simulink model "Googol_XY_machine_test"  (R2020a)
settings: Solver=ode14x  StartTime=0.0  StopTime=15  RelTol=1e-3  EnableMultiTasking=on
values from neighbouring files (symbols this model uses):
  N = length(signal)    [plotfft.m]    (also in script_cascade.m = length(out_with.cascade.signals(2).values); script_pid.m = length(out_with.PID.signals(2).values))
  new_kd = gains(1)    [script.m]    (also in script_pid.m)
  new_ki = gains(3)    [script.m]    (also in script_pid.m)
  new_kp = gains(2)    [script.m]    (also in script_pid.m)
undefined symbols (not defined in the file or in its folder): X, Y, Z
libraries: sm_lib x10, simulink x8, nesl_utility x7
settings Model: Creator=Admin  LastModifiedBy=Admin
settings SolverCC: AutoInsertRateTranBlk=on
settings DataIOCC: LimitDataPoints=on  MaxDataPoints=10000  ReturnWorkspaceOutputsName=out_without
settings OptimizationCC: LifeSpan=inf
settings DebuggingCC: AllowSymbolicDim=off  SFUnexpectedBacktrackingDiag=warning  SFNoUnconditionalDefaultTransitionDiag=warning  SFExecutionAtInitializationDiag=none  ArithmeticOperatorsInVariantConditions=warning
settings SFSimCC: SimUseLocalCustomCode=off  CustomCodeUndefinedFunction=UseInterfaceOnly
settings RTWCC: RTWUseLocalCustomCode=off
settings CodeAppCC: StateflowObjectComments=on
settings GRTTargetCC: TargetLangStandard=C89/C90 (ANSI)
settings ConfigComp: CovMetricSettings=dw  CovHtmlReporting=on  CovSaveCumulativeToWorkspaceVar=on  CovSaveSingleToWorkspaceVar=on  CovExternalEMLEnable=off  CovSFcnEnable=off
settings SimscapeCC: SimscapeLogType=all  SimscapeLogSimulationStatistics=on  SimscapeLogDataHistory=10000

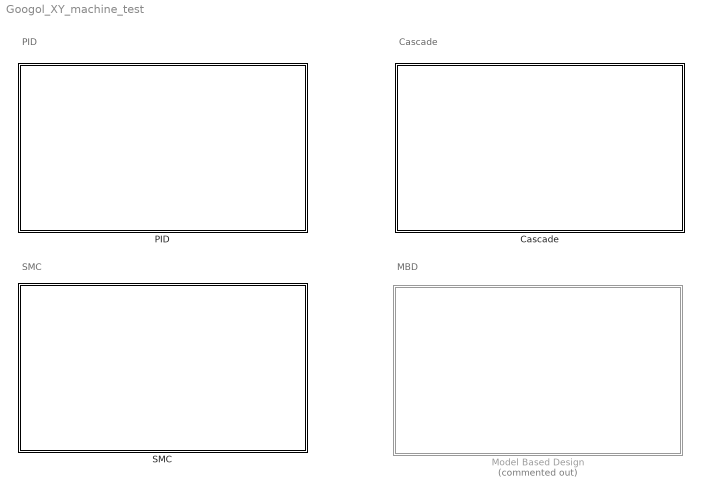
== system Googol_XY_machine_test ==
  note: MBD
  note: Cascade
  note: PID
  note: SMC
  Cascade : Subsystem
  Model Based Design : Subsystem  Commented=on
  PID : Subsystem
  SMC : Subsystem

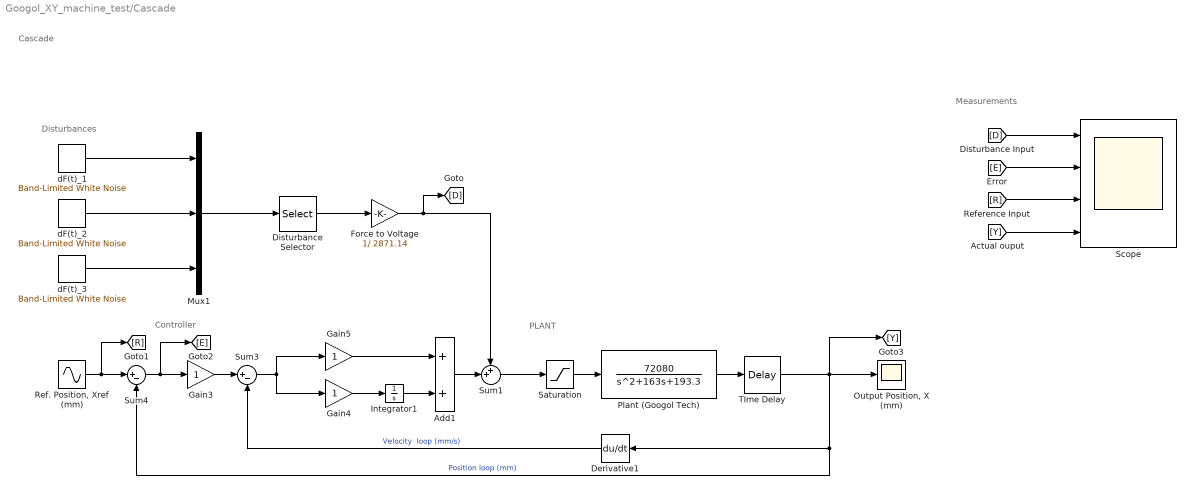
== system Googol_XY_machine_test/Cascade ==
  note: PLANT
  note: Controller
  note: Measurements
  note: Disturbances
  note: Cascade
  Add1 : Sum
  Derivative1 : Derivative
  Disturbance Selector : Selector  InputPortWidth=3  IndexOptions=Index vector (dialog)  Indices=[1]  OutputSizes=1
  Force to Voltage : Gain  Gain=1/ 2871.14
  Gain3 : Gain
  Gain4 : Gain
  Gain5 : Gain
  Integrator1 : Integrator  InitialCondition=.1
  Mux1 : Mux  Inputs=3
  "Output Position, X (mm)" : Scope
  Plant (Googol Tech) : TransferFcn  Numerator=[72080]  Denominator=[1 163 193.3]
  "Ref. Position, Xref (mm)" : Sin  SampleTime=0
  Saturation : Saturate  UpperLimit=92  LowerLimit=-92
  Scope : Scope  NumInputPorts=4
  Sum1 : Sum  Inputs=++|
  Sum3 : Sum  Inputs=|+-
  Sum4 : Sum  Inputs=|+-
  TIme Delay : TransportDelay  DelayTime=0.0012
  dF(t)_1 : simulink/Sources/Band-Limited White Noise  Cov=[0.1]  Ts=5e-4  seed=[23341]
  dF(t)_2 : simulink/Sources/Band-Limited White Noise  Cov=[0.1]  Ts=0.1  seed=[23341]
  dF(t)_3 : simulink/Sources/Band-Limited White Noise  Cov=[0.1]  Ts=0.1  seed=[23341]
  wires:
  dF(t)_3/1 -> Mux1/3
  TIme Delay/1 -> "Output Position, X (mm)"/1, [Y], Derivative1/1, Sum4/2  "Position loop (mm)"
  Sum1/1 -> Saturation/1
  Gain5/1 -> Add1/1
  Integrator1/1 -> Add1/2
  Plant (Googol Tech)/1 -> TIme Delay/1
  Sum3/1 -> Gain5/1, Gain4/1
  "Ref. Position, Xref (mm)"/1 -> Sum4/1, [R]
  Sum4/1 -> Gain3/1, [E]
  Derivative1/1 -> Sum3/2  "Velocity  loop (mm/s)"
  Gain3/1 -> Sum3/1
  Disturbance Selector/1 -> Force to Voltage/1
  Gain4/1 -> Integrator1/1
  Add1/1 -> Sum1/2
  dF(t)_2/1 -> Mux1/2
  dF(t)_1/1 -> Mux1/1
  Mux1/1 -> Disturbance Selector/1
  Force to Voltage/1 -> Sum1/1, [D]
  [D] -> Scope/1
  [E] -> Scope/2
  [R] -> Scope/3
  [Y] -> Scope/4
  Saturation/1 -> Plant (Googol Tech)/1

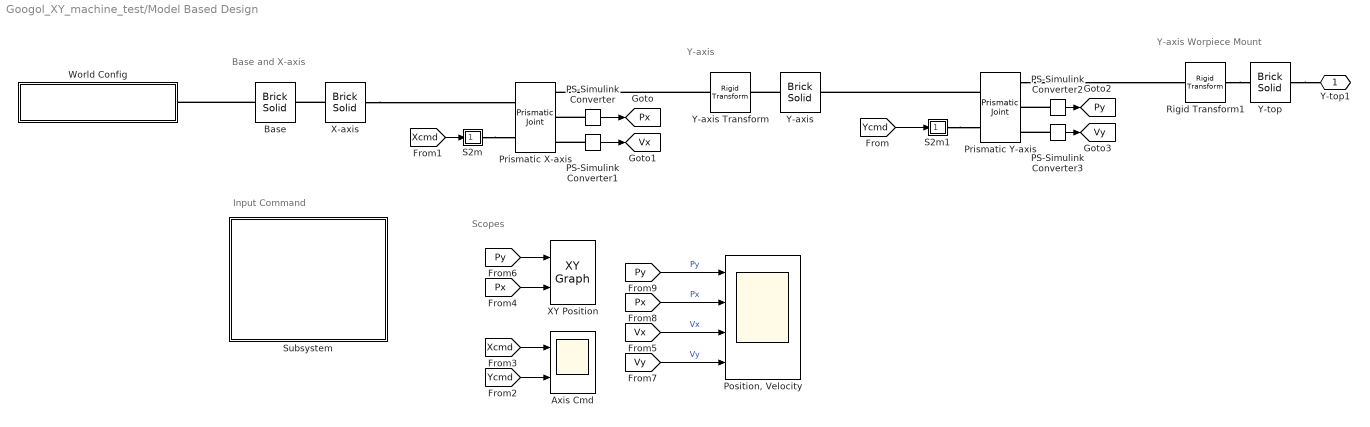
== system Googol_XY_machine_test/Model Based Design ==
  note: Input Command
  note: Scopes
  note: Base and X-axis
  note: Y-axis
  note: Y-axis Worpiece Mount
  Axis Cmd : Scope  NumInputPorts=2
  Base : sm_lib/Body Elements/Brick Solid  GraphicAmbientColor=[0.15 0.15 0.15 1.0]  BasedOnType=Density  BrickDimensions=[630 470 10]  BrickDimensionUnits=mm  CenterOfMass=[0 0 0]  CenterOfMassUnits=m  GraphicDiffuseColor=[0.4 0.4 0.4]  Density=1000  DensityUnits=kg/m^3  DoExposeReferenceFrame=on  GraphicEmissiveColor=[0.0 0.0 0.0 1.0]  ExportEntireGeometry=off  SerializedFrames=<Frames><Frame><Id>Frame1</Id><Value><Name>F1</Name><Origin><Source>GeometricFeature</Source><FeatureName>+z surface</FeatureName></Origin><PrimaryAxis><DefinedDirection>+Z</DefinedDirection><Source>ReferenceFrame</Source><SourceDirection>+Z</SourceDirection><FeatureName></FeatureName></PrimaryAxis><SecondaryAxis><DefinedDirection>+X</DefinedDirection><Source>ReferenceFrame</Source><SourceDirection>+X</SourceDirection><FeatureName></FeatureName></SecondaryAxis></Value></Frame></Frames>  MarkerShape=Sphere  MarkerSize=10  GraphicType=FromGeometry  InertiaType=CalculateFromGeometry  Mass=1  MassUnits=kg  MomentsOfInertia=[1 1 1]  MomentsOfInertiaUnits=kg*m^2  GraphicOpacity=1.0  ProductsOfInertia=[0 0 0]  ProductsOfInertiaUnits=kg*m^2  GraphicShininess=75  GraphicSpecularColor=[0.5 0.5 0.5 1.0]  GraphicVisPropType=SimpleVisualProperties
  PS-Simulink Converter : nesl_utility/PS-Simulink Converter  PhysicalDomain=network_engine_domain  SubClassName=ps_output  LeftPortType=input  RightPortType=output  PseudoPeriodic=off  Frequencies=[]  Unit=mm  AffineConversion=off
  PS-Simulink Converter1 : nesl_utility/PS-Simulink Converter  PhysicalDomain=network_engine_domain  SubClassName=ps_output  LeftPortType=input  RightPortType=output  PseudoPeriodic=off  Frequencies=[]  Unit=m/s  AffineConversion=off
  PS-Simulink Converter2 : nesl_utility/PS-Simulink Converter  PhysicalDomain=network_engine_domain  SubClassName=ps_output  LeftPortType=input  RightPortType=output  PseudoPeriodic=off  Frequencies=[]  Unit=mm  AffineConversion=off
  PS-Simulink Converter3 : nesl_utility/PS-Simulink Converter  PhysicalDomain=network_engine_domain  SubClassName=ps_output  LeftPortType=input  RightPortType=output  PseudoPeriodic=off  Frequencies=[]  Unit=m/s  AffineConversion=off
  "Position, Velocity" : Scope  NumInputPorts=4
  Prismatic X-axis : sm_lib/Joints/Prismatic Joint  JointMode=Normal  SenseConstraintForce=off  SenseConstraintForceX=off  SenseConstraintForceY=off  SenseConstraintForceZ=off  SenseConstraintTorque=off  SenseConstraintTorqueX=off  SenseConstraintTorqueY=off  SenseConstraintTorqueZ=off  SenseTotalForce=off  SenseTotalForceX=off  SenseTotalForceY=off  SenseTotalForceZ=off  SenseTotalTorque=off  SenseTotalTorqueX=off  SenseTotalTorqueY=off  SenseTotalTorqueZ=off  CompositeWrenchDir=FollowerOnBase  CompositeWrenchFrame=BaseFrame  EquilibriumPosition=0  EquilibriumPositionUnits=m  SpringStiffness=0  SpringStiffnessUnits=N/m  DampingCoefficient=0  DampingCoefficientUnits=N/(m/s)  TorqueActuationMode=ComputedTorque  MotionActuationMode=InputMotion  SensePosition=on  SenseVelocity=on  SenseAcceleration=off  SenseTorqueForce=off  SenseLowerLimitTorqueForce=off  SenseUpperLimitTorqueForce=off  LowerLimitSpecify=on  LowerLimitBound=-115  LowerLimitBoundUnits=mm  LowerLimitStiffness=1e3  LowerLimitStiffnessUnits=N/m  LowerLimitDamping=1e3  LowerLimitDampingUnits=N/(m/s)  LowerLimitTransitionRegionWidth=1e-4  LowerLimitTransitionRegionWidthUnits=m  UpperLimitSpecify=on  UpperLimitBound=115  UpperLimitBoundUnits=mm  UpperLimitStiffness=1e3  UpperLimitStiffnessUnits=N/m  UpperLimitDamping=1e3  UpperLimitDampingUnits=N/(m/s)  UpperLimitTransitionRegionWidth=1e-4  UpperLimitTransitionRegionWidthUnits=m  PositionTargetSpecify=off  PositionTargetPriority=High  PositionTargetValue=0  PositionTargetValueUnits=m  VelocityTargetSpecify=off  VelocityTargetPriority=High  VelocityTargetValue=0  VelocityTargetValueUnits=m/s
  Prismatic Y-axis : sm_lib/Joints/Prismatic Joint  JointMode=Normal  SenseConstraintForce=off  SenseConstraintForceX=off  SenseConstraintForceY=off  SenseConstraintForceZ=off  SenseConstraintTorque=off  SenseConstraintTorqueX=off  SenseConstraintTorqueY=off  SenseConstraintTorqueZ=off  SenseTotalForce=off  SenseTotalForceX=off  SenseTotalForceY=off  SenseTotalForceZ=off  SenseTotalTorque=off  SenseTotalTorqueX=off  SenseTotalTorqueY=off  SenseTotalTorqueZ=off  CompositeWrenchDir=FollowerOnBase  CompositeWrenchFrame=BaseFrame  EquilibriumPosition=0  EquilibriumPositionUnits=m  SpringStiffness=0  SpringStiffnessUnits=N/m  DampingCoefficient=0  DampingCoefficientUnits=N/(m/s)  TorqueActuationMode=ComputedTorque  MotionActuationMode=InputMotion  SensePosition=on  SenseVelocity=on  SenseAcceleration=off  SenseTorqueForce=off  SenseLowerLimitTorqueForce=off  SenseUpperLimitTorqueForce=off  LowerLimitSpecify=on  LowerLimitBound=-115  LowerLimitBoundUnits=mm  LowerLimitStiffness=10  LowerLimitStiffnessUnits=N/m  LowerLimitDamping=1e3  LowerLimitDampingUnits=N/(m/s)  LowerLimitTransitionRegionWidth=1e-4  LowerLimitTransitionRegionWidthUnits=m  UpperLimitSpecify=on  UpperLimitBound=115  UpperLimitBoundUnits=mm  UpperLimitStiffness=10  UpperLimitStiffnessUnits=N/m  UpperLimitDamping=1e3  UpperLimitDampingUnits=N/(m/s)  UpperLimitTransitionRegionWidth=1e-4  UpperLimitTransitionRegionWidthUnits=m  PositionTargetSpecify=off  PositionTargetPriority=High  PositionTargetValue=0  PositionTargetValueUnits=m  VelocityTargetSpecify=off  VelocityTargetPriority=High  VelocityTargetValue=0  VelocityTargetValueUnits=m/s
  Rigid Transform1 : sm_lib/Frames and Transforms/Rigid Transform  TranslationMethod=None  TranslationStandardOffset=0  TranslationLengthUnit=m  TranslationStandardAxis=+Z  TranslationCartesianOffset=[0 0 0]  TranslationROffset=0  TranslationROffsetUnits=m  TranslationZOffset=0  TranslationZOffsetUnits=m  TranslationThetaOffset=0  TranslationThetaOffsetUnits=deg  RotationMethod=StandardAxis  RotationAngleUnits=deg  RotationStandardAxis=+Y  RotationAngle=-90  RotationArbitraryAxis=[0 0 1]  FollAlignAxisA=+X  BaseAlignAxisA=+Y  FollAlignAxisB=+Y  BaseAlignAxisB=+Z  RotationSequenceAxes=FollowerAxes  RotationSequence=XYX  RotationSequenceAngles=[0 0 0]  RotationSequenceAnglesUnits=deg  RotationMatrix=[1 0 0; 0 1 0; 0 0 1]
  S2m : Subsystem
  S2m1 : Subsystem
  Subsystem : Subsystem  mask{ax=0.044, ay=0.046, Fx=0.540, Fy=0.510}
      mask prompts: ax "Amplitude_X"; ay "Amplitude_Y"; Fx "Frequency_X"; Fy "Frequency_Y"
      mask DialogControl DescTextVar Prompt: Tune different motion parameters, Amplitude, a and Frequency, f
      mask DialogControl Container12 Prompt: Amplitude
      mask DialogControl Container13 Prompt: Frequency
      mask DialogControl Container3 Prompt: FREQUENCY
      mask Display: image('$imagefile'); % Use "Edit Image" on toolstrip to change.
  World Config : Subsystem
  X-axis : sm_lib/Body Elements/Brick Solid  GraphicAmbientColor=[0.15 0.15 0.15 1.0]  BasedOnType=Density  BrickDimensions=[70 300 40]  BrickDimensionUnits=mm  CenterOfMass=[0 0 0]  CenterOfMassUnits=m  GraphicDiffuseColor=[0.2 0.6 1.0]  Density=1000  DensityUnits=kg/m^3  DoExposeReferenceFrame=off  GraphicEmissiveColor=[0.0 0.0 0.0 1.0]  ExportEntireGeometry=off  SerializedFrames=<Frames><Frame><Id>Frame1</Id><Value><Name>F1</Name><Origin><Source>GeometricFeature</Source><FeatureName>+z surface</FeatureName></Origin><PrimaryAxis><DefinedDirection>+Z</DefinedDirection><Source>ReferenceFrame</Source><SourceDirection>-Y</SourceDirection><FeatureName></FeatureName></PrimaryAxis><SecondaryAxis><DefinedDirection>+X</DefinedDirection><Source>ReferenceFrame</Source><SourceDirection>+X</SourceDirection><FeatureName></FeatureName></SecondaryAxis></Value></Frame><Frame><Id>Frame2</Id><Value><Name>F2</Name><Origin><Source>GeometricFeature</Source><FeatureName>-z surface</FeatureName></Origin><PrimaryAxis><DefinedDirection>+Z</DefinedDirection><Source>ReferenceFrame</Source><SourceDirection>+Z</SourceDirection><FeatureName></FeatureName></PrimaryAxis><SecondaryAxis><DefinedDirection>+X</DefinedDirection><Source>ReferenceFrame</Source><SourceDirection>+X</SourceDirection><FeatureName></FeatureName></SecondaryAxis></Value></Frame></Frames>  MarkerShape=Sphere  MarkerSize=10  GraphicType=FromGeometry  InertiaType=CalculateFromGeometry  Mass=1  MassUnits=kg  MomentsOfInertia=[1 1 1]  MomentsOfInertiaUnits=kg*m^2  GraphicOpacity=1.0  ProductsOfInertia=[0 0 0]  ProductsOfInertiaUnits=kg*m^2  GraphicShininess=75  GraphicSpecularColor=[0.5 0.5 0.5 1.0]  GraphicVisPropType=SimpleVisualProperties
  XY Position : simulink/Sinks/XY Graph  xmin=-300  xmax=300  ymin=-300  ymax=300  st=.1
  Y-axis : sm_lib/Body Elements/Brick Solid  GraphicAmbientColor=[0.15 0.15 0.15 1.0]  BasedOnType=Density  BrickDimensions=[300 70 40]  BrickDimensionUnits=mm  CenterOfMass=[0 0 0]  CenterOfMassUnits=m  GraphicDiffuseColor=[0.8 0.6 0.0]  Density=1000  DensityUnits=kg/m^3  DoExposeReferenceFrame=off  GraphicEmissiveColor=[0.0 0.0 0.0 1.0]  ExportEntireGeometry=off  SerializedFrames=<Frames><Frame><Id>Frame1</Id><Value><Name>F1</Name><Origin><Source>GeometricFeature</Source><FeatureName>+z surface</FeatureName></Origin><PrimaryAxis><DefinedDirection>+Z</DefinedDirection><Source>ReferenceFrame</Source><SourceDirection>+X</SourceDirection><FeatureName></FeatureName></PrimaryAxis><SecondaryAxis><DefinedDirection>+Y</DefinedDirection><Source>ReferenceFrame</Source><SourceDirection>+Y</SourceDirection><FeatureName></FeatureName></SecondaryAxis></Value></Frame><Frame><Id>Frame2</Id><Value><Name>F2</Name><Origin><Source>GeometricFeature</Source><FeatureName>-z surface</FeatureName></Origin><PrimaryAxis><DefinedDirection>+Z</DefinedDirection><Source>ReferenceFrame</Source><SourceDirection>+Z</SourceDirection><FeatureName></FeatureName></PrimaryAxis><SecondaryAxis><DefinedDirection>+X</DefinedDirection><Source>ReferenceFrame</Source><SourceDirection>+X</SourceDirection><FeatureName></FeatureName></SecondaryAxis></Value></Frame></Frames>  MarkerShape=Sphere  MarkerSize=10  GraphicType=FromGeometry  InertiaType=CalculateFromGeometry  Mass=1  MassUnits=kg  MomentsOfInertia=[1 1 1]  MomentsOfInertiaUnits=kg*m^2  GraphicOpacity=1.0  ProductsOfInertia=[0 0 0]  ProductsOfInertiaUnits=kg*m^2  GraphicShininess=75  GraphicSpecularColor=[0.5 0.5 0.5 1.0]  GraphicVisPropType=SimpleVisualProperties
  Y-axis Transform : sm_lib/Frames and Transforms/Rigid Transform  TranslationMethod=None  TranslationStandardOffset=0  TranslationLengthUnit=m  TranslationStandardAxis=+Z  TranslationCartesianOffset=[0 0 0]  TranslationROffset=0  TranslationROffsetUnits=m  TranslationZOffset=0  TranslationZOffsetUnits=m  TranslationThetaOffset=0  TranslationThetaOffsetUnits=deg  RotationMethod=StandardAxis  RotationAngleUnits=deg  RotationStandardAxis=+X  RotationAngle=-90  RotationArbitraryAxis=[0 0 1]  FollAlignAxisA=+X  BaseAlignAxisA=+Y  FollAlignAxisB=+Y  BaseAlignAxisB=+Z  RotationSequenceAxes=FollowerAxes  RotationSequence=XYX  RotationSequenceAngles=[0 0 0]  RotationSequenceAnglesUnits=deg  RotationMatrix=[1 0 0; 0 1 0; 0 0 1]
  Y-top : sm_lib/Body Elements/Brick Solid  GraphicAmbientColor=[0.15 0.15 0.15 1.0]  BasedOnType=Density  BrickDimensions=[70 70 10]  BrickDimensionUnits=mm  CenterOfMass=[0 0 0]  CenterOfMassUnits=m  GraphicDiffuseColor=[0.2 0.2 0.2]  Density=1000  DensityUnits=kg/m^3  DoExposeReferenceFrame=off  GraphicEmissiveColor=[0.0 0.0 0.0 1.0]  ExportEntireGeometry=off  SerializedFrames=<Frames><Frame><Id>Frame1</Id><Value><Name>F1</Name><Origin><Source>GeometricFeature</Source><FeatureName>+z surface</FeatureName></Origin><PrimaryAxis><DefinedDirection>+Z</DefinedDirection><Source>ReferenceFrame</Source><SourceDirection>+Z</SourceDirection><FeatureName></FeatureName></PrimaryAxis><SecondaryAxis><DefinedDirection>+X</DefinedDirection><Source>ReferenceFrame</Source><SourceDirection>+X</SourceDirection><FeatureName></FeatureName></SecondaryAxis></Value></Frame><Frame><Id>Frame2</Id><Value><Name>F2</Name><Origin><Source>GeometricFeature</Source><FeatureName>-z surface</FeatureName></Origin><PrimaryAxis><DefinedDirection>+Z</DefinedDirection><Source>ReferenceFrame</Source><SourceDirection>+Z</SourceDirection><FeatureName></FeatureName></PrimaryAxis><SecondaryAxis><DefinedDirection>+X</DefinedDirection><Source>ReferenceFrame</Source><SourceDirection>+X</SourceDirection><FeatureName></FeatureName></SecondaryAxis></Value></Frame></Frames>  MarkerShape=Sphere  MarkerSize=10  GraphicType=FromGeometry  InertiaType=CalculateFromGeometry  Mass=1  MassUnits=kg  MomentsOfInertia=[1 1 1]  MomentsOfInertiaUnits=kg*m^2  GraphicOpacity=1.0  ProductsOfInertia=[0 0 0]  ProductsOfInertiaUnits=kg*m^2  GraphicShininess=75  GraphicSpecularColor=[0.5 0.5 0.5 1.0]  GraphicVisPropType=SimpleVisualProperties
  Y-top1 : PMIOPort  Side=Left
  tag scope: Px=global, Py=global, Vx=global, Vy=global
  wires:
  [Px] -> XY Position/2
  PS-Simulink Converter1/1 -> [Vx]
  [Ycmd] -> Axis Cmd/2
  [Ycmd] -> S2m1/1(In)
  [Xcmd] -> S2m/1(In)
  PS-Simulink Converter2/1 -> [Py]
  PS-Simulink Converter3/1 -> [Vy]
  PS-Simulink Converter/1 -> [Px]
  [Py] -> "Position, Velocity"/1  "Py"
  [Vy] -> "Position, Velocity"/4  "Vy"
  [Py] -> XY Position/1
  [Vx] -> "Position, Velocity"/3  "Vx"
  [Px] -> "Position, Velocity"/2  "Px"
  [Xcmd] -> Axis Cmd/1
  connections:
  Y-axis/RConn1 -- Y-axis Transform/RConn1
  PS-Simulink Converter2/LConn1 -- Prismatic Y-axis/RConn2
  PS-Simulink Converter1/LConn1 -- Prismatic X-axis/RConn3
  Y-axis Transform/LConn1 -- Prismatic X-axis/RConn1
  Prismatic Y-axis/RConn1 -- Rigid Transform1/LConn1
  S2m1/RConn1 -- Prismatic Y-axis/LConn2
  Base/RConn1 -- World Config/RConn1
  Rigid Transform1/RConn1 -- Y-top/RConn1
  Prismatic Y-axis/LConn1 -- Y-axis/LConn1
  X-axis/LConn1 -- Prismatic X-axis/LConn1
  S2m/RConn1 -- Prismatic X-axis/LConn2
  PS-Simulink Converter3/LConn1 -- Prismatic Y-axis/RConn3
  PS-Simulink Converter/LConn1 -- Prismatic X-axis/RConn2
  X-axis/RConn1 -- Base/LConn1
  Y-top/LConn1 -- Y-top1/RConn1

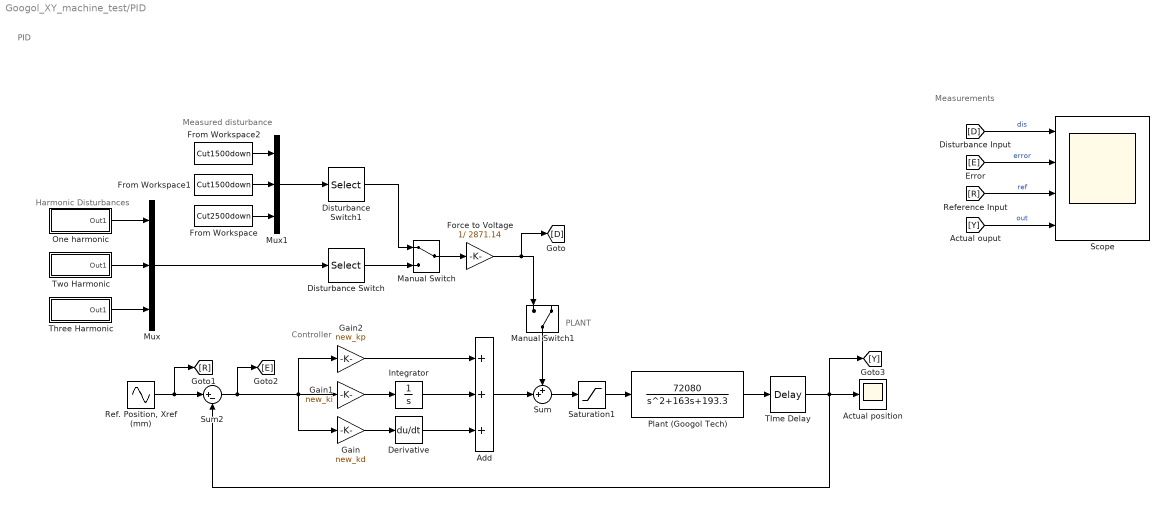
== system Googol_XY_machine_test/PID ==
  note: Measured disturbance
  note: PID
  note: Harmonic Disturbances
  note: Controller
  note: PLANT
  note: Measurements
  Actual position : Scope
  Add : Sum  Inputs=+++
  Derivative : Derivative
  Disturbance Switch : Selector  InputPortWidth=3  IndexOptions=Index vector (dialog)  Indices=[2]  OutputSizes=1
  Disturbance Switch1 : Selector  InputPortWidth=3  IndexOptions=Index vector (dialog)  Indices=[1]  OutputSizes=1
  Force to Voltage : Gain  Gain=1/ 2871.14
  From Workspace : FromWorkspace  VariableName=Cut2500down  OutputAfterFinalValue=Setting to zero
  From Workspace1 : FromWorkspace  VariableName=Cut1500down  OutDataTypeStr=double  OutputAfterFinalValue=Setting to zero
  From Workspace2 : FromWorkspace  VariableName=Cut1500down  OutDataTypeStr=double  OutputAfterFinalValue=Setting to zero
  Gain : Gain  Gain=new_kd
  Gain1 : Gain  Gain=new_ki
  Gain2 : Gain  Gain=new_kp
  Integrator : Integrator
  Manual Switch : ManualSwitch
  Manual Switch1 : ManualSwitch  CurrentSetting=0
  Mux : Mux  Inputs=3
  Mux1 : Mux  Inputs=3
  One harmonic : Subsystem
  Plant (Googol Tech) : TransferFcn  Numerator=[72080]  Denominator=[1 163 193.3]
  "Ref. Position, Xref (mm)" : Sin  Amplitude=5  Frequency=0.5*(2*pi)  SampleTime=0  Offset=1/2000
  Saturation1 : Saturate  UpperLimit=92  LowerLimit=-92
  Scope : Scope  NumInputPorts=4
  Sum : Sum  Inputs=++|
  Sum2 : Sum  Inputs=|+-
  TIme Delay : TransportDelay  DelayTime=0.0012
  Three Harmonic : Subsystem
  Two Harmonic : Subsystem
  wires:
  Gain1/1 -> Integrator/1
  Gain2/1 -> Add/1
  TIme Delay/1 -> [Y], Sum2/2, Actual position/1
  "Ref. Position, Xref (mm)"/1 -> [R], Sum2/1
  Derivative/1 -> Add/3
  Sum2/1 -> [E], Gain/1, Gain1/1, Gain2/1
  Integrator/1 -> Add/2
  Gain/1 -> Derivative/1
  Two Harmonic/1(Out1) -> Mux/2
  Add/1 -> Sum/2
  One harmonic/1(Out1) -> Mux/1
  Plant (Googol Tech)/1 -> TIme Delay/1
  Three Harmonic/1(Out1) -> Mux/3
  Sum/1 -> Saturation1/1
  Mux/1 -> Disturbance Switch/1
  Force to Voltage/1 -> Manual Switch1/1, [D]
  [R] -> Scope/3  "ref"
  [E] -> Scope/2  "error"
  [Y] -> Scope/4  "out"
  [D] -> Scope/1  "dis"
  Disturbance Switch/1 -> Manual Switch/2
  Manual Switch/1 -> Force to Voltage/1
  Saturation1/1 -> Plant (Googol Tech)/1
  From Workspace2/1 -> Mux1/1
  From Workspace1/1 -> Mux1/2
  From Workspace/1 -> Mux1/3
  Mux1/1 -> Disturbance Switch1/1
  Manual Switch1/1 -> Sum/1
  Disturbance Switch1/1 -> Manual Switch/1

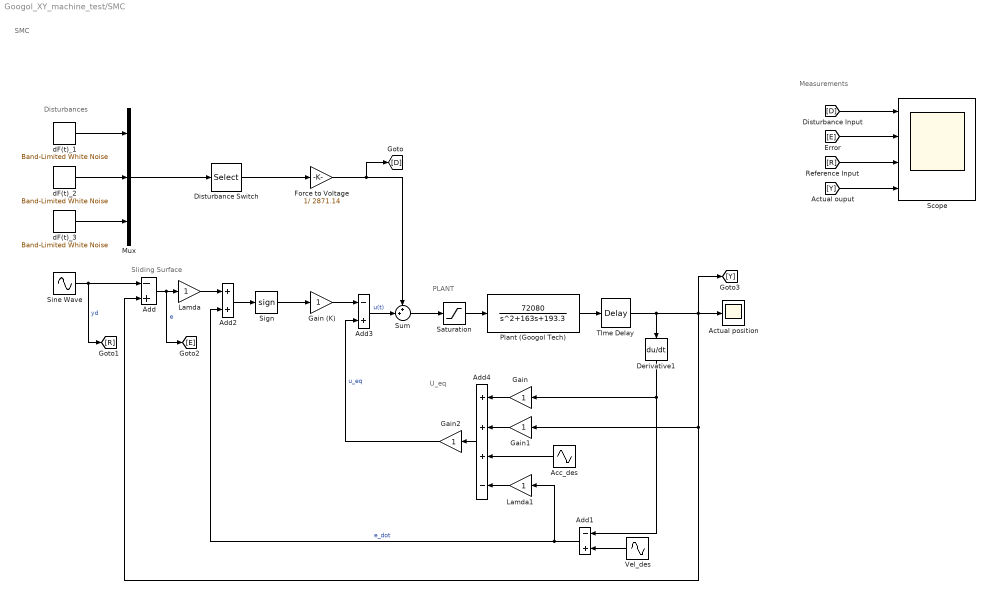
== system Googol_XY_machine_test/SMC ==
  note: Sliding Surface
  note: U_eq
  note: Measurements
  note: PLANT
  note: Disturbances
  note: SMC
  Acc_des : Sin  SampleTime=0
  Actual position : Scope
  Add : Sum  Inputs=-+
  Add1 : Sum  Inputs=-+
  Add2 : Sum
  Add3 : Sum  Inputs=-+
  Add4 : Sum  Inputs=+++-
  Derivative1 : Derivative
  Disturbance Switch : Selector  InputPortWidth=3  IndexOptions=Index vector (dialog)  Indices=[2]  OutputSizes=1
  Force to Voltage : Gain  Gain=1/ 2871.14
  Gain : Gain
  Gain (K) : Gain
  Gain1 : Gain
  Gain2 : Gain
  Lamda : Gain
  Lamda1 : Gain
  Mux : Mux  Inputs=3
  Plant (Googol Tech) : TransferFcn  Numerator=[72080]  Denominator=[1 163 193.3]
  Saturation : Saturate  UpperLimit=92  LowerLimit=-92
  Scope : Scope  NumInputPorts=4
  Sign : Signum
  Sine Wave : Sin  SampleTime=0
  Sum : Sum  Inputs=++|
  TIme Delay : TransportDelay  DelayTime=0.0012
  Vel_des : Sin  SampleTime=0
  dF(t)_1 : simulink/Sources/Band-Limited White Noise  Cov=[0.1]  Ts=5e-4  seed=[23341]
  dF(t)_2 : simulink/Sources/Band-Limited White Noise  Cov=[0.1]  Ts=0.1  seed=[23341]
  dF(t)_3 : simulink/Sources/Band-Limited White Noise  Cov=[0.1]  Ts=0.1  seed=[23341]
  wires:
  [D] -> Scope/1
  [Y] -> Scope/4
  [E] -> Scope/2
  [R] -> Scope/3
  Force to Voltage/1 -> Sum/1, [D]
  Mux/1 -> Disturbance Switch/1
  Saturation/1 -> Plant (Googol Tech)/1
  dF(t)_3/1 -> Mux/3
  Plant (Googol Tech)/1 -> TIme Delay/1
  Sum/1 -> Saturation/1
  dF(t)_1/1 -> Mux/1
  dF(t)_2/1 -> Mux/2
  Disturbance Switch/1 -> Force to Voltage/1
  Sine Wave/1 -> Add/1, [R]  "yd"
  Add/1 -> [E], Lamda/1  "e"
  Lamda/1 -> Add2/1
  TIme Delay/1 -> [Y], Actual position/1, Add/2, Gain1/1, Derivative1/1
  Sign/1 -> Gain (K)/1
  Vel_des/1 -> Add1/2
  Add1/1 -> Add2/2, Lamda1/1  "e_dot"
  Add2/1 -> Sign/1
  Gain (K)/1 -> Add3/1
  Gain2/1 -> Add3/2  "u_eq"
  Add3/1 -> Sum/2  "u(t)"
  Derivative1/1 -> Add1/1, Gain/1
  Gain/1 -> Add4/1
  Gain1/1 -> Add4/2
  Acc_des/1 -> Add4/3
  Lamda1/1 -> Add4/4
  Add4/1 -> Gain2/1

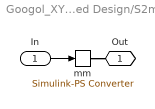
== system Googol_XY_machine_test/Model Based Design/S2m ==
  In : Inport
  mm : nesl_utility/Simulink-PS Converter  PhysicalDomain=network_engine_domain  SubClassName=ps_input  LeftPortType=input  RightPortType=output  PseudoPeriodic=off  Frequencies=[]  NoiseDistribution=none  NoiseParameters=[]  Unit=mm  AffineConversion=off  FilteringAndDerivatives=filter  SimscapeFilterOrder=2  InputFilterTimeConstant=0.001  UdotUserProvided=0
      settings: SourceProductBaseCode=MT,SS
  Out : PMIOPort  Side=Right
  wires:
  In/1 -> mm/1
  connections:
  mm/RConn1 -- Out/RConn1

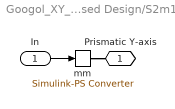
== system Googol_XY_machine_test/Model Based Design/S2m1 ==
  In : Inport
  mm : nesl_utility/Simulink-PS Converter  PhysicalDomain=network_engine_domain  SubClassName=ps_input  LeftPortType=input  RightPortType=output  PseudoPeriodic=off  Frequencies=[]  NoiseDistribution=none  NoiseParameters=[]  Unit=mm  AffineConversion=off  FilteringAndDerivatives=filter  SimscapeFilterOrder=2  InputFilterTimeConstant=0.001  UdotUserProvided=0
      settings: SourceProductBaseCode=MT,SS
  Prismatic Y-axis : PMIOPort  Side=Right
  wires:
  In/1 -> mm/1
  connections:
  mm/RConn1 -- Prismatic Y-axis/RConn1

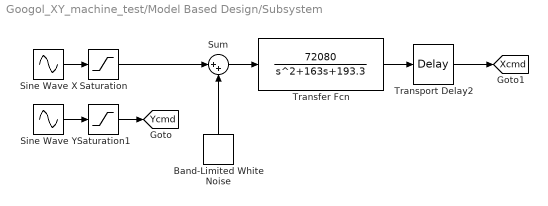
== system Googol_XY_machine_test/Model Based Design/Subsystem ==
  Band-Limited White Noise : simulink/Sources/Band-Limited White Noise  Cov=[1e-5]  Ts=0.1  seed=[23341]
  Saturation : Saturate  UpperLimit=.2  LowerLimit=-.2
  Saturation1 : Saturate  UpperLimit=.1  LowerLimit=-.1
  Sine Wave X : Sin  Amplitude=ax  Frequency=Fx  SampleTime=0
  Sine Wave Y : Sin  Amplitude=ay  Frequency=Fy  Phase=8  SampleTime=0
  Sum : Sum  Inputs=|++
  Transfer Fcn : TransferFcn  Numerator=[72080]  Denominator=[1 163 193.3]
  Transport Delay2 : TransportDelay  DelayTime=0.0012
  tag scope: Xcmd=global, Ycmd=global
  wires:
  Saturation1/1 -> [Ycmd]
  Sine Wave X/1 -> Saturation/1
  Sine Wave Y/1 -> Saturation1/1
  Band-Limited White Noise/1 -> Sum/2
  Transfer Fcn/1 -> Transport Delay2/1
  Sum/1 -> Transfer Fcn/1
  Transport Delay2/1 -> [Xcmd]
  Saturation/1 -> Sum/1

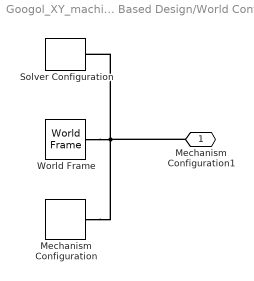
== system Googol_XY_machine_test/Model Based Design/World Config ==
  Mechanism Configuration : sm_lib/Utilities/Mechanism Configuration  UniformGravity=Constant  GravityVector=[0 0 -9.80665]  GravityUnits=m/s^2  LinearizationDelta=0.001
  Solver Configuration : nesl_utility/Solver Configuration  PhysicalDomain=network_engine_domain  SubClassName=solver  LeftPortType=input  RightPortType=generic  Tones=[]  Harmonics=[]  SimulateNoise=off  Profile=off  UseLocalSampling=off  EnableSwitchedLinearOptims=on  FrequencyDomain=off  UseCCode=off  RelTol=0.001  AbsTol=1e-06  MinStep=1e-09  ToWorkspace=off  RevertToSquareIcSolve=off  NumHomotopyIterations=100  PhasorMode=off  PhasorModeNumHarmonics=1  DoDC=off  ResidualTolerance=1e-09  UseLocalSolver=off  LocalSolverChoice=NE_BACKWARD_EULER_ADVANCER  LocalSolverSampleTime=0.001  DoFixedCost=off  MaxNonlinIter=3  MaxModeIter=2  LinearAlgebra=Sparse  EquationFormulation=NE_TIME_EF  DelaysMemoryBudget=1024  AutomaticFiltering=on  FilteringTimeConstant=0.001  PartitionStorageMethod=AS_NEEDED  PartitionMemoryBudget=1024  PartitionMethod=FAST
      settings: SourceProductBaseCode=MT,SS
  World Frame : sm_lib/Frames and Transforms/World Frame
  Mechanism Configuration1 : PMIOPort  Side=Right
  connections:
  World Frame/RConn1 -- Mechanism Configuration1/RConn1 -- Solver Configuration/RConn1 -- Mechanism Configuration/RConn1

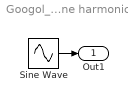
== system Googol_XY_machine_test/PID/One harmonic ==
  Sine Wave : Sin  Amplitude=0.5  Frequency=0.2*2*pi  SampleTime=0
  Out1 : Outport
  wires:
  Sine Wave/1 -> Out1/1

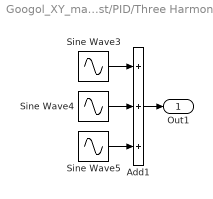
== system Googol_XY_machine_test/PID/Three Harmonic ==
  Add1 : Sum  Inputs=+++
  Sine Wave3 : Sin  Amplitude=0.2  Frequency=0.2*2*pi  SampleTime=0
  Sine Wave4 : Sin  Amplitude=0.2  Frequency=0.5*2*pi  SampleTime=0
  Sine Wave5 : Sin  Amplitude=0.2  Frequency=0.8*2*pi  SampleTime=0
  Out1 : Outport
  wires:
  Sine Wave3/1 -> Add1/1
  Sine Wave5/1 -> Add1/3
  Sine Wave4/1 -> Add1/2
  Add1/1 -> Out1/1

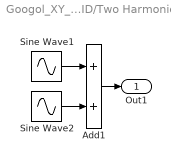
== system Googol_XY_machine_test/PID/Two Harmonic ==
  Add1 : Sum
  Sine Wave1 : Sin  Amplitude=0.3  Frequency=0.2*2*pi  SampleTime=0
  Sine Wave2 : Sin  Amplitude=0.3  Frequency=0.5*2*pi  SampleTime=0
  Out1 : Outport
  wires:
  Sine Wave2/1 -> Add1/2
  Sine Wave1/1 -> Add1/1
  Add1/1 -> Out1/1
